simulink subsystem "In_Plane_Model"  (R2025b)
settings: Solver=VariableStepAuto  StartTime=0.0  StopTime=10.0  RelTol=1e-3
undefined symbols (not defined in the file): AeroLiftCff, AeroLongDrgCff, AeroMotoEffctArea, AeroPitchMomentCff, AeroPitchMomentLngth, AeroRltWindAngVect, AeroSideFrcCff, AeroYawMomentCff, aMode, BrkFrntBrkActrBore, BrkFrntBrkActrPrsBpt, BrkFrntBrkPadMeanRadius, BrkFrntBrkTrqTbl, BrkFrntIntrnRadius, BrkFrntKinFricCff, BrkFrntPadNum, BrkFrntShoePinToDrumCntrDst, BrkFrntShoePinToFrcAppDst, BrkFrntShoePinToPadEndAng, BrkFrntShoePinToPadStartAng, BrkFrntStcFricCff, BrkFrntWhlSpdBpt, BrkRearBrkActrBore, BrkRearBrkActrPrsBpt, BrkRearBrkPadMeanRadius, BrkRearBrkTrqTbl, BrkRearIntrnRadius, BrkRearKinFricCff, BrkRearPadNum, BrkRearShoePinToDrumCntrDst, BrkRearShoePinToFrcAppDst, BrkRearShoePinToPadEndAng, BrkRearShoePinToPadStartAng, BrkRearStcFricCff, BrkRearWhlSpdBpt, EnvAbsPrs, EnvAirTemp, FrkFrL0, FrmAng0, g, GasCnst, InitFrkLngth, InitMainFrmPitchAng, InitRearArmPitchAng, InitRearCntctPtchLatVel, InitRearCntctPtchLongVel, InitRearCntctPtchY, InitRearCntctPtchZ, InitRollAng, InitYawAng, MotoFrmLngth, MotoFrmMass, MotoGrvty, MotoLatOfst, MotoLongOfst, MotoLowrFrntFrkMass, MotoPtchOfst, MotoRearArmLngth, MotoRearArmMass, MotoRollOfst ... (+25)
libraries: sm_lib x309, nesl_utility_internal x158, nesl_utility x7, autolibsharedcoupling x6, vehdynlibtire x6, sharedtransform x4, shared6dof x1, matrix_library x1, vehdynlibeomcommon x1
(part 3 of 10)

== system In_Plane_Model/Chassis, Tires, and Areo/Chassis Body, Suspension, and Steering/CHASSIS/Chassis body/JointHubRr ==
  Bus Creator : BusCreator  Inputs=3
  PS-Simulink Converter3 : nesl_utility_internal/PS-Simulink Converter  PhysicalDomain=network_engine_domain  SubClassName=ps_output  LeftPortType=input  RightPortType=output  PseudoPeriodic=off  Frequencies=[]  VectorFormat=1-D array  Unit=inherit  AffineConversion=off
  PS-Simulink Converter4 : nesl_utility_internal/PS-Simulink Converter  PhysicalDomain=network_engine_domain  SubClassName=ps_output  LeftPortType=input  RightPortType=output  PseudoPeriodic=off  Frequencies=[]  VectorFormat=1-D array  Unit=inherit  AffineConversion=off
  PS-Simulink Converter8 : nesl_utility_internal/PS-Simulink Converter  PhysicalDomain=network_engine_domain  SubClassName=ps_output  LeftPortType=input  RightPortType=output  PseudoPeriodic=off  Frequencies=[]  VectorFormat=1-D array  Unit=inherit  AffineConversion=off
  Pitch dof : sm_lib/Joints/Revolute Joint  JointMode=Normal  CompositeWrenchDir=FollowerOnBase  CompositeWrenchFrame=BaseFrame  SenseConstraintForce=off  SenseConstraintTorque=off  SenseTotalForce=off  SenseTotalTorque=off  PositionTargetSpecify=on  PositionTargetPriority=High  PositionTargetValue=InitRearArmPitchAng  PositionTargetValueUnits=rad  VelocityTargetSpecify=on  VelocityTargetPriority=High  VelocityTargetValue=InitRearArmPitchRate  VelocityTargetValueUnits=rad/s  EquilibriumPosition=0  EquilibriumPositionUnits=rad  SpringStiffness=0  SpringStiffnessUnits=N*m/rad  DampingCoefficient=0  DampingCoefficientUnits=N*m/(rad/s)  LowerLimitSpecify=off  LowerLimitBound=-90  LowerLimitBoundUnits=deg  LowerLimitStiffness=1e4  LowerLimitStiffnessUnits=N*m/deg  LowerLimitDamping=10  LowerLimitDampingUnits=N*m/(deg/s)  LowerLimitTransitionRegionWidth=0.1  LowerLimitTransitionRegionWidthUnits=deg  UpperLimitSpecify=off  UpperLimitBound=90  UpperLimitBoundUnits=deg  UpperLimitStiffness=1e4  UpperLimitStiffnessUnits=N*m/deg  UpperLimitDamping=10  UpperLimitDampingUnits=N*m/(deg/s)  UpperLimitTransitionRegionWidth=0.1  UpperLimitTransitionRegionWidthUnits=deg  TorqueActuationMode=NoTorque  MotionActuationMode=ComputedMotion  SensePosition=on  SenseVelocity=on  SenseAcceleration=on  SenseTorqueForce=off  SenseLowerLimitTorqueForce=off  SenseUpperLimitTorqueForce=off
  World vertical frame : Subsystem  VariantControl=World vertical
  X_-pi/2 : sm_lib/Frames and Transforms/Rigid Transform  RotationMethod=StandardAxis  FollAlignAxisA=+X  BaseAlignAxisA=+Y  FollAlignAxisB=+Y  BaseAlignAxisB=+Z  RotationStandardAxis=+X  RotationAngle=-pi/2  RotationAngleUnits=rad  RotationArbitraryAxis=[0 0 1]  RotationSequenceAxes=FollowerAxes  RotationSequence=XYX  RotationSequenceAngles=[0 0 0]  RotationSequenceAnglesUnits=deg  RotationMatrix=[1 0 0; 0 1 0; 0 0 1]  Quaternion=[1 0 0 0]  TranslationMethod=None  TranslationCartesianOffset=[0 0 0]  TranslationCartesianOffsetUnits=m  TranslationStandardAxis=+Z  TranslationStandardOffset=0  TranslationStandardOffsetUnits=m  TranslationROffset=0  TranslationROffsetUnits=m  TranslationThetaOffset=0  TranslationThetaOffsetUnits=deg  TranslationZOffset=0  TranslationZOffsetUnits=m
  X_pi/2 : sm_lib/Frames and Transforms/Rigid Transform  RotationMethod=StandardAxis  FollAlignAxisA=+X  BaseAlignAxisA=+Y  FollAlignAxisB=+Y  BaseAlignAxisB=+Z  RotationStandardAxis=+X  RotationAngle=pi/2  RotationAngleUnits=rad  RotationArbitraryAxis=[0 0 1]  RotationSequenceAxes=FollowerAxes  RotationSequence=XYX  RotationSequenceAngles=[0 0 0]  RotationSequenceAnglesUnits=deg  RotationMatrix=[1 0 0; 0 1 0; 0 0 1]  Quaternion=[1 0 0 0]  TranslationMethod=None  TranslationCartesianOffset=[0 0 0]  TranslationCartesianOffsetUnits=m  TranslationStandardAxis=+Z  TranslationStandardOffset=0  TranslationStandardOffsetUnits=m  TranslationROffset=0  TranslationROffsetUnits=m  TranslationThetaOffset=0  TranslationThetaOffsetUnits=deg  TranslationZOffset=0  TranslationZOffsetUnits=m
  F : PMIOPort  Side=Left
  WVFrame_WhlRr : PMIOPort  Port=2  Side=Left
  B : PMIOPort  Port=3  Side=Right
  A,V,P : Outport
  wires:
  PS-Simulink Converter8/1 -> Bus Creator/2  "ArmRrAngV"
  Bus Creator/1 -> A,V,P/1  "ArmRrAng"
  PS-Simulink Converter3/1 -> Bus Creator/1  "ArmRrAngA"
  PS-Simulink Converter4/1 -> Bus Creator/3  "ArmRrAng"
  connections:
  WVFrame_WhlRr/RConn1 -- World vertical frame/RConn1
  X_pi/2/LConn1 -- Pitch dof/RConn1
  PS-Simulink Converter8/LConn1 -- Pitch dof/RConn3
  PS-Simulink Converter3/LConn1 -- Pitch dof/RConn4
  PS-Simulink Converter4/LConn1 -- Pitch dof/RConn2
  X_-pi/2/LConn1 -- B/RConn1
  F/RConn1 -- World vertical frame/LConn1 -- X_pi/2/RConn1
  Pitch dof/LConn1 -- X_-pi/2/RConn1

== system In_Plane_Model/Chassis, Tires, and Areo/Chassis Body, Suspension, and Steering/CHASSIS/Chassis body/Origin&Env ==
  Course shape : Subsystem  Variant=on  VariantControlMode=label  VariantControl=Choice  LabelModeActiveChoice=none
  Ground : Subsystem  Commented=on
  Inertial Frame : sm_lib/Body Elements/Graphic  Commented=on  GraphicType=Marker  MarkerShape=Frame  MarkerSize=30  GraphicVisPropType=SimpleVisualProperties  GraphicDiffuseColor=[0.0 0.0 0.0]  GraphicOpacity=1.0  GraphicSpecularColor=[0.5 0.5 0.5 1.0]  GraphicAmbientColor=[0.15 0.15 0.15 1.0]  GraphicEmissiveColor=[0.0 0.0 0.0 1.0]  GraphicShininess=75
  Mechanism Configuration : sm_lib/Utilities/Mechanism Configuration  UniformGravity=Constant  GravityVector=[-MotoGrvty*sin(0) 0 -MotoGrvty*cos(0)]  GravityVectorUnits=m/s^2  LinearizationDelta=0.001  JointModeTransitionNonlinearIterations=2
  Solver Configuration : nesl_utility_internal/Solver Configuration  PhysicalDomain=network_engine_domain  SubClassName=solver  LeftPortType=input  RightPortType=generic  Tones=[]  Harmonics=[]  SimulateNoise=off  Profile=off  UseLocalSampling=off  EnableSwitchedLinearOptims=on  FrequencyDomain=off  UseCCode=off  RelTol=0.001  AbsTol=1e-06  MinStep=1e-09  ToWorkspace=off  RevertToSquareIcSolve=off  NumHomotopyIterations=100  PhasorMode=off  PhasorModeNumHarmonics=1  ConsistencySolver=NEWTON_FTOL  IndexReductionMethod=DerivativeReplacement  DoDC=off  ResidualTolerance=1e-3  ConsistencyTolSource=GLOBAL  ConsistencyAbsTol=0.001  ConsistencyRelTol=0.001  ConsistencyTolFactor=0.001  UseLocalSolver=on  LocalSolverChoice=NE_BACKWARD_EULER_ADVANCER  ResolveIndetEquations=on  FunctionEvalNumThread=1  LocalSolverSampleTime=0.01  DoFixedCost=off  MaxNonlinIter=3  MaxModeIter=2  ComputeImpulses=off  ImpulseIterations=2  LinearAlgebra=Sparse  LinearAlgebraNumThread=0  EquationFormulation=NE_TIME_EF  DelaysMemoryBudget=1024  AutomaticFiltering=on  FilteringTimeConstant=0.001  PartitionStorageMethod=AS_NEEDED  PartitionMemoryBudget=1024  PartitionMethod=FAST  MultibodyUseLocalSolver=on  MultibodyLocalSolverChoice=ODE1  MultibodyLocalSolverSampleTime=0.01
  World Frame : sm_lib/Frames and Transforms/World Frame
  setSAE : sm_lib/Frames and Transforms/Rigid Transform  RotationMethod=StandardAxis  FollAlignAxisA=+X  BaseAlignAxisA=+Y  FollAlignAxisB=+Y  BaseAlignAxisB=+Z  RotationStandardAxis=+X  RotationAngle=pi  RotationAngleUnits=rad  RotationArbitraryAxis=[0 0 1]  RotationSequenceAxes=FollowerAxes  RotationSequence=XYX  RotationSequenceAngles=[0 0 0]  RotationSequenceAnglesUnits=deg  RotationMatrix=[1 0 0; 0 1 0; 0 0 1]  Quaternion=[1 0 0 0]  TranslationMethod=None  TranslationCartesianOffset=[0 0 0]  TranslationCartesianOffsetUnits=m  TranslationStandardAxis=+Z  TranslationStandardOffset=0  TranslationStandardOffsetUnits=m  TranslationROffset=0  TranslationROffsetUnits=m  TranslationThetaOffset=0  TranslationThetaOffsetUnits=deg  TranslationZOffset=0  TranslationZOffsetUnits=m
  F : PMIOPort  Side=Left
  connections:
  setSAE/RConn1 -- F/RConn1 -- Inertial Frame/RConn1
  Course shape/LConn1 -- Ground/LConn1 -- setSAE/LConn1 -- Solver Configuration/RConn1 -- Mechanism Configuration/RConn1 -- World Frame/RConn1

== system In_Plane_Model/Chassis, Tires, and Areo/Chassis Body, Suspension, and Steering/CHASSIS/Chassis body/mass_ArmRr ==
  CGCoord. : sm_lib/Frames and Transforms/Rigid Transform  RotationMethod=None  FollAlignAxisA=+X  BaseAlignAxisA=+Y  FollAlignAxisB=+Y  BaseAlignAxisB=+Z  RotationStandardAxis=+X  RotationAngle=0  RotationAngleUnits=rad  RotationArbitraryAxis=[0 0 1]  RotationSequenceAxes=FollowerAxes  RotationSequence=XYX  RotationSequenceAngles=[0 0 0]  RotationSequenceAnglesUnits=deg  RotationMatrix=[1 0 0; 0 1 0; 0 0 1]  Quaternion=[1 0 0 0]  TranslationMethod=Cartesian  TranslationCartesianOffset=MotoRearArmPos  TranslationCartesianOffsetUnits=m  TranslationStandardAxis=+X  TranslationStandardOffset=0  TranslationStandardOffsetUnits=m  TranslationROffset=0  TranslationROffsetUnits=m  TranslationThetaOffset=0  TranslationThetaOffsetUnits=deg  TranslationZOffset=0  TranslationZOffsetUnits=m
  CG_Solid : sm_lib/Body Elements/Spherical Solid  SphereRadius=3e-2  SphereRadiusUnits=m  ExportEntireGeometry=off  InertiaType=Custom  BasedOnType=Density  Density=1000  DensityUnits=kg/m^3  Mass=MotoRearArmMass  MassUnits=kg  CenterOfMass=[0 0 0]  CenterOfMassUnits=m  MomentsOfInertia=MotoRearArmInert  MomentsOfInertiaUnits=kg*m^2  ProductsOfInertia=[0 0 0]  ProductsOfInertiaUnits=kg*m^2  GraphicType=FromGeometry  MarkerShape=Sphere  MarkerSize=10  GraphicVisPropType=SimpleVisualProperties  GraphicDiffuseColor=[1.0 0.0 0.0]  GraphicOpacity=1.0  GraphicSpecularColor=[0.5 0.5 0.5 1.0]  GraphicAmbientColor=[0.15 0.15 0.15 1.0]  GraphicEmissiveColor=[0.0 0.0 0.0 1.0]  GraphicShininess=75  DoExposeReferenceFrame=on  SerializedFrames=<Frames/>
  Graphic : sm_lib/Body Elements/Graphic  GraphicType=Marker  MarkerShape=Frame  MarkerSize=30  GraphicVisPropType=SimpleVisualProperties  GraphicDiffuseColor=[0.0 0.0 1.0]  GraphicOpacity=1.0  GraphicSpecularColor=[0.5 0.5 0.5 1.0]  GraphicAmbientColor=[0.15 0.15 0.15 1.0]  GraphicEmissiveColor=[0.0 0.0 0.0 1.0]  GraphicShininess=75
  World vertical frame : Subsystem  VariantControl=World vertical
  B : PMIOPort  Side=Left
  CG : PMIOPort  Port=2  Side=Right
  WVFrame_ArmRr : PMIOPort  Port=3  Side=Right
  connections:
  WVFrame_ArmRr/RConn1 -- World vertical frame/RConn1
  Graphic/RConn1 -- B/RConn1 -- CGCoord./LConn1
  CG/RConn1 -- CGCoord./RConn1 -- World vertical frame/LConn1 -- CG_Solid/RConn1

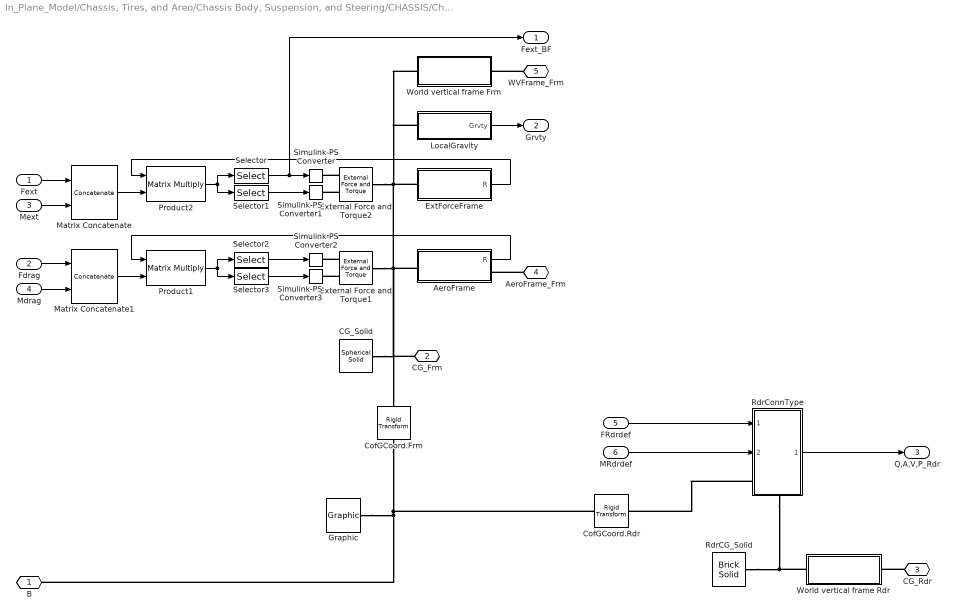
== system In_Plane_Model/Chassis, Tires, and Areo/Chassis Body, Suspension, and Steering/CHASSIS/Chassis body/mass_Frm ==
  Fext : Inport
  Fdrag : Inport  Port=2
  Mext : Inport  Port=3
  Mdrag : Inport  Port=4
  FRdrdef : Inport  Port=5
  MRdrdef : Inport  Port=6
  AeroFrame : Subsystem  Variant=on  VariantControlMode=label  VariantControl=Choice  LabelModeActiveChoice=World vertical
  CG_Solid : sm_lib/Body Elements/Spherical Solid  SphereRadius=3e-2  SphereRadiusUnits=m  ExportEntireGeometry=off  InertiaType=Custom  BasedOnType=Density  Density=1000  DensityUnits=kg/m^3  Mass=MotoFrmMass  MassUnits=kg  CenterOfMass=[0 0 0]  CenterOfMassUnits=m  MomentsOfInertia=MotoFrmInert  MomentsOfInertiaUnits=kg*m^2  ProductsOfInertia=[0 0 0]  ProductsOfInertiaUnits=kg*m^2  GraphicType=FromGeometry  MarkerShape=Sphere  MarkerSize=10  GraphicVisPropType=SimpleVisualProperties  GraphicDiffuseColor=[1.0 0.0 0.0]  GraphicOpacity=1.0  GraphicSpecularColor=[0.5 0.5 0.5 1.0]  GraphicAmbientColor=[0.15 0.15 0.15 1.0]  GraphicEmissiveColor=[0.0 0.0 0.0 1.0]  GraphicShininess=75  DoExposeReferenceFrame=on  SerializedFrames=<Frames/>
  CofGCoord.Frm : sm_lib/Frames and Transforms/Rigid Transform  RotationMethod=None  FollAlignAxisA=+X  BaseAlignAxisA=+Y  FollAlignAxisB=+Y  BaseAlignAxisB=+Z  RotationStandardAxis=+X  RotationAngle=0  RotationAngleUnits=rad  RotationArbitraryAxis=[0 0 1]  RotationSequenceAxes=FollowerAxes  RotationSequence=XYX  RotationSequenceAngles=[0 0 0]  RotationSequenceAnglesUnits=deg  RotationMatrix=[1 0 0; 0 1 0; 0 0 1]  Quaternion=[1 0 0 0]  TranslationMethod=Cartesian  TranslationCartesianOffset=MotoFrmCm  TranslationCartesianOffsetUnits=m  TranslationStandardAxis=+X  TranslationStandardOffset=0  TranslationStandardOffsetUnits=m  TranslationROffset=0  TranslationROffsetUnits=m  TranslationThetaOffset=0  TranslationThetaOffsetUnits=deg  TranslationZOffset=0  TranslationZOffsetUnits=m
  CofGCoord.Rdr : sm_lib/Frames and Transforms/Rigid Transform  RotationMethod=None  FollAlignAxisA=+X  BaseAlignAxisA=+Y  FollAlignAxisB=+Y  BaseAlignAxisB=+Z  RotationStandardAxis=+X  RotationAngle=0  RotationAngleUnits=rad  RotationArbitraryAxis=[0 0 1]  RotationSequenceAxes=FollowerAxes  RotationSequence=XYX  RotationSequenceAngles=[0 0 0]  RotationSequenceAnglesUnits=deg  RotationMatrix=[1 0 0; 0 1 0; 0 0 1]  Quaternion=[1 0 0 0]  TranslationMethod=Cartesian  TranslationCartesianOffset=RiderCmLoct  TranslationCartesianOffsetUnits=m  TranslationStandardAxis=+X  TranslationStandardOffset=0  TranslationStandardOffsetUnits=m  TranslationROffset=0  TranslationROffsetUnits=m  TranslationThetaOffset=0  TranslationThetaOffsetUnits=deg  TranslationZOffset=0  TranslationZOffsetUnits=m
  ExtForceFrame : Subsystem  Variant=on  VariantControlMode=label  VariantControl=Choice  LabelModeActiveChoice=World vertical
  External Force and Torque1 : sm_lib/Forces and Torques/External Force and Torque  EnableForceX=off  EnableForceY=off  EnableForceZ=off  EnableForce=on  ForceResolutionFrame=AttachedFrame  EnableTorqueX=off  EnableTorqueY=off  EnableTorqueZ=off  EnableTorque=on  TorqueResolutionFrame=AttachedFrame
  External Force and Torque2 : sm_lib/Forces and Torques/External Force and Torque  EnableForceX=off  EnableForceY=off  EnableForceZ=off  EnableForce=on  ForceResolutionFrame=AttachedFrame  EnableTorqueX=off  EnableTorqueY=off  EnableTorqueZ=off  EnableTorque=on  TorqueResolutionFrame=AttachedFrame
  Graphic : sm_lib/Body Elements/Graphic  GraphicType=Marker  MarkerShape=Frame  MarkerSize=30  GraphicVisPropType=SimpleVisualProperties  GraphicDiffuseColor=[0.0 0.0 1.0]  GraphicOpacity=1.0  GraphicSpecularColor=[0.5 0.5 0.5 1.0]  GraphicAmbientColor=[0.15 0.15 0.15 1.0]  GraphicEmissiveColor=[0.0 0.0 0.0 1.0]  GraphicShininess=75
  LocalGravity : Subsystem
  Matrix Concatenate : Concatenate  Mode=Multidimensional array  ConcatenateDimension=2
  Matrix Concatenate1 : Concatenate  Mode=Multidimensional array  ConcatenateDimension=2
  Product1 : Product  Multiplication=Matrix(*)
  Product2 : Product  Multiplication=Matrix(*)
  RdrCG_Solid : sm_lib/Body Elements/Brick Solid  BrickDimensions=[1 1 1]*0.1  BrickDimensionsUnits=m  ExportEntireGeometry=off  InertiaType=Custom  BasedOnType=Density  Density=1000  DensityUnits=kg/m^3  Mass=RiderMass  MassUnits=kg  CenterOfMass=[0 0 0]  CenterOfMassUnits=m  MomentsOfInertia=RiderInert  MomentsOfInertiaUnits=kg*m^2  ProductsOfInertia=[0 0 0]  ProductsOfInertiaUnits=kg*m^2  GraphicType=FromGeometry  MarkerShape=Sphere  MarkerSize=10  GraphicVisPropType=SimpleVisualProperties  GraphicDiffuseColor=[0.4 0.4 0.4]  GraphicOpacity=1.0  GraphicSpecularColor=[0.5 0.5 0.5 1.0]  GraphicAmbientColor=[0.15 0.15 0.15 1.0]  GraphicEmissiveColor=[0.0 0.0 0.0 1.0]  GraphicShininess=75  DoExposeReferenceFrame=on  SerializedFrames=<Frames/>
  RdrConnType : Subsystem  Variant=on  VariantChoicesSpecifier={'Rigid', 's6DOF_and_External_Forces_and_Moments'}  VariantControlMode=label  VariantControl=Choice  LabelModeActiveChoice=Rigid
      settings: PortSchema="{\"entries\":[{\"content\":{\"sides\":[{\"content\":{\"connectorIds\":[\"In1\",\"In2\",\"LConn1\"]},\"type\":\"ConnectorPlacement.EquallySpacedRectSide\",\"uuid\":\"6027bf0c-47dc-4641-b312-91f0cbb185cc\"},{\"content\":{\"connectorIds\":[\"Out1\"],\"side\":\"RIGHT\"},\"type\":\"ConnectorPlacement.EquallySpacedRectSide\",\"uuid\":\"75561f8d-b6fc-4ce9-bdf9-6e985548130f\"},{\"content\":{\"side\":\"TOP\"},\"type\":\"ConnectorPlacement.EquallySpacedRectSide\",\"uuid\":\"398f9736-f514-4440-baa3-55debf119b8f\"},{\"content\":{\"connectorIds\":[\"RConn1\"],\"side\":\"BOTTOM\"},\"type\":\"ConnectorPlacement.EquallySpacedRectSide\",\"uuid\":\"dfd8777e-2555-41c1-b77e-3f19d71f018f\"}]},\"type\":\"ConnectorPlacement.EquallySpacedConnector\",\"uuid\":\"9426d2e3-04b5-4679-a13c-19ca1f9bfd84\"}],\"packageUris\":[\"http://schema.mathworks.com/mf0/Connector/R2020b\"],\"version\":\"1.0\"}"
  Selector : Selector  NumberOfDimensions=2  InputPortWidth=3  IndexOptions=Index vector (dialog),Index vector (dialog)  Indices=[1 2 3],[1]  OutputSizes=1,1
  Selector1 : Selector  NumberOfDimensions=2  InputPortWidth=3  IndexOptions=Index vector (dialog),Index vector (dialog)  Indices=[1 2 3],[2]  OutputSizes=1,1
  Selector2 : Selector  NumberOfDimensions=2  InputPortWidth=3  IndexOptions=Index vector (dialog),Index vector (dialog)  Indices=[1 2 3],[1]  OutputSizes=1,1
  Selector3 : Selector  NumberOfDimensions=2  InputPortWidth=3  IndexOptions=Index vector (dialog),Index vector (dialog)  Indices=[1 2 3],[2]  OutputSizes=1,1
  Simulink-PS Converter : nesl_utility_internal/Simulink-PS Converter  PhysicalDomain=network_engine_domain  SubClassName=ps_input  LeftPortType=input  RightPortType=output  PseudoPeriodic=off  Frequencies=[]  NoiseDistribution=none  NoiseParameters=[]  Unit=N  AffineConversion=off  FilteringAndDerivatives=provide  SimscapeFilterOrder=1  InputFilterTimeConstant=0.001  UdotUserProvided=0
  Simulink-PS Converter1 : nesl_utility_internal/Simulink-PS Converter  PhysicalDomain=network_engine_domain  SubClassName=ps_input  LeftPortType=input  RightPortType=output  PseudoPeriodic=off  Frequencies=[]  NoiseDistribution=none  NoiseParameters=[]  Unit=N*m  AffineConversion=off  FilteringAndDerivatives=provide  SimscapeFilterOrder=1  InputFilterTimeConstant=0.001  UdotUserProvided=0
  Simulink-PS Converter2 : nesl_utility_internal/Simulink-PS Converter  PhysicalDomain=network_engine_domain  SubClassName=ps_input  LeftPortType=input  RightPortType=output  PseudoPeriodic=off  Frequencies=[]  NoiseDistribution=none  NoiseParameters=[]  Unit=N  AffineConversion=off  FilteringAndDerivatives=provide  SimscapeFilterOrder=1  InputFilterTimeConstant=0.001  UdotUserProvided=0
  Simulink-PS Converter3 : nesl_utility_internal/Simulink-PS Converter  PhysicalDomain=network_engine_domain  SubClassName=ps_input  LeftPortType=input  RightPortType=output  PseudoPeriodic=off  Frequencies=[]  NoiseDistribution=none  NoiseParameters=[]  Unit=N*m  AffineConversion=off  FilteringAndDerivatives=provide  SimscapeFilterOrder=1  InputFilterTimeConstant=0.001  UdotUserProvided=0
  World vertical frame Frm : Subsystem  VariantControl=World vertical
  World vertical frame Rdr : Subsystem  VariantControl=World vertical
  B : PMIOPort  Side=Left
  CG_Frm : PMIOPort  Port=2  Side=Right
  CG_Rdr : PMIOPort  Port=3  Side=Right
  AeroFrame_Frm : PMIOPort  Port=4  Side=Right
  WVFrame_Frm : PMIOPort  Port=5  Side=Right
  Fext_BF : Outport
  Grvty : Outport  Port=2
  Q,A,V,P_Rdr : Outport  Port=3
  wires:
  FRdrdef/1 -> RdrConnType/1(FRdrdef)
  MRdrdef/1 -> RdrConnType/2(MRdrdef)
  RdrConnType/1(Q,A,V,P_Rdr) -> Q,A,V,P_Rdr/1
  AeroFrame/1(R) -> Product1/1
  Fdrag/1 -> Matrix Concatenate1/1
  Mdrag/1 -> Matrix Concatenate1/2
  Selector3/1 -> Simulink-PS Converter3/1
  Matrix Concatenate1/1 -> Product1/2
  Product1/1 -> Selector3/1, Selector2/1
  Selector2/1 -> Simulink-PS Converter2/1
  LocalGravity/1(Grvty) -> Grvty/1
  Selector/1 -> Fext_BF/1, Simulink-PS Converter/1
  Product2/1 -> Selector/1, Selector1/1
  Matrix Concatenate/1 -> Product2/2
  Selector1/1 -> Simulink-PS Converter1/1
  Mext/1 -> Matrix Concatenate/2
  Fext/1 -> Matrix Concatenate/1
  ExtForceFrame/1(R) -> Product2/1
  connections:
  CG_Rdr/RConn1 -- World vertical frame Rdr/RConn1
  WVFrame_Frm/RConn1 -- World vertical frame Frm/RConn1
  AeroFrame_Frm/RConn1 -- AeroFrame/RConn1
  RdrConnType/LConn1 -- CofGCoord.Rdr/RConn1
  World vertical frame Rdr/LConn1 -- RdrConnType/RConn1 -- RdrCG_Solid/RConn1
  External Force and Torque1/LConn1 -- Simulink-PS Converter2/RConn1
  External Force and Torque1/LConn2 -- Simulink-PS Converter3/RConn1
  ExtForceFrame/LConn1 -- External Force and Torque1/RConn1 -- AeroFrame/LConn1 -- CG_Frm/RConn1 -- CofGCoord.Frm/RConn1 -- CG_Solid/RConn1 -- LocalGravity/LConn1 -- World vertical frame Frm/LConn1 -- External Force and Torque2/RConn1
  External Force and Torque2/LConn2 -- Simulink-PS Converter1/RConn1
  External Force and Torque2/LConn1 -- Simulink-PS Converter/RConn1
  CofGCoord.Frm/LConn1 -- CofGCoord.Rdr/LConn1 -- B/RConn1 -- Graphic/RConn1

== system In_Plane_Model/Chassis, Tires, and Areo/Chassis Body, Suspension, and Steering/CHASSIS/Chassis body/pivo (dofPitch) ==
  MSusr : Inport
  Bus Creator : BusCreator  Inputs=3
  Selector : Selector  InputPortWidth=3  IndexOptions=Index vector (dialog)  Indices=3  OutputSizes=1
  pivo : Subsystem  Variant=on  VariantControlMode=label  VariantControl=Choice  LabelModeActiveChoice=pivo
  B : PMIOPort  Side=Left
  F : PMIOPort  Port=2  Side=Left
  A,V,P : Outport
  My : Outport  Port=2
  wires:
  MSusr/1 -> pivo/1(t)
  Bus Creator/1 -> A,V,P/1  "FrmAng"
  pivo/1(q) -> Bus Creator/3  "FrmAng"
  pivo/3(b) -> Bus Creator/1  "FrmAngA"
  pivo/2(w) -> Bus Creator/2  "FrmAngV"
  Selector/1 -> My/1  "MsuspRr"
  pivo/4(tt) -> Selector/1
  connections:
  pivo/RConn1 -- F/RConn1
  pivo/LConn1 -- B/RConn1

== system In_Plane_Model/Chassis, Tires, and Areo/Chassis Body, Suspension, and Steering/CHASSIS/Sensors/Geom sensor ==
  Bus Creator : BusCreator  Inputs=12
  Graphic1 : sm_lib/Body Elements/Graphic  GraphicType=Marker  MarkerShape=Frame  MarkerSize=20  GraphicVisPropType=SimpleVisualProperties  GraphicDiffuseColor=[1 1 0]  GraphicOpacity=1.0  GraphicSpecularColor=[0.5 0.5 0.5 1.0]  GraphicAmbientColor=[0.15 0.15 0.15 1.0]  GraphicEmissiveColor=[0.0 0.0 0.0 1.0]  GraphicShininess=75
  Graphic2 : sm_lib/Body Elements/Graphic  GraphicType=Marker  MarkerShape=Frame  MarkerSize=20  GraphicVisPropType=SimpleVisualProperties  GraphicDiffuseColor=[1 1 0]  GraphicOpacity=1.0  GraphicSpecularColor=[0.5 0.5 0.5 1.0]  GraphicAmbientColor=[0.15 0.15 0.15 1.0]  GraphicEmissiveColor=[0.0 0.0 0.0 1.0]  GraphicShininess=75
  Graphic3 : sm_lib/Body Elements/Graphic  GraphicType=Marker  MarkerShape=Frame  MarkerSize=20  GraphicVisPropType=SimpleVisualProperties  GraphicDiffuseColor=[1 1 0]  GraphicOpacity=1.0  GraphicSpecularColor=[0.5 0.5 0.5 1.0]  GraphicAmbientColor=[0.15 0.15 0.15 1.0]  GraphicEmissiveColor=[0.0 0.0 0.0 1.0]  GraphicShininess=75
  Sensor_HubFr : Subsystem
  Sensor_HubRr : Subsystem
  Sensor_origin : Subsystem
  UE4orig2HubFr : sm_lib/Frames and Transforms/Rigid Transform  RotationMethod=None  FollAlignAxisA=+X  BaseAlignAxisA=+Y  FollAlignAxisB=+Y  BaseAlignAxisB=+Z  RotationStandardAxis=+X  RotationAngle=0  RotationAngleUnits=rad  RotationArbitraryAxis=[0 0 1]  RotationSequenceAxes=FollowerAxes  RotationSequence=XYX  RotationSequenceAngles=[0 0 0]  RotationSequenceAnglesUnits=deg  RotationMatrix=[1 0 0; 0 1 0; 0 0 1]  Quaternion=[1 0 0 0]  TranslationMethod=Cartesian  TranslationCartesianOffset=[ScnFrntHubX, 0, ScnFrntHubZ]  TranslationCartesianOffsetUnits=m  TranslationStandardAxis=+X  TranslationStandardOffset=0  TranslationStandardOffsetUnits=m  TranslationROffset=0  TranslationROffsetUnits=m  TranslationThetaOffset=0  TranslationThetaOffsetUnits=deg  TranslationZOffset=0  TranslationZOffsetUnits=m
  UE4orig2HubRr : sm_lib/Frames and Transforms/Rigid Transform  RotationMethod=None  FollAlignAxisA=+X  BaseAlignAxisA=+Y  FollAlignAxisB=+Y  BaseAlignAxisB=+Z  RotationStandardAxis=+X  RotationAngle=0  RotationAngleUnits=rad  RotationArbitraryAxis=[0 0 1]  RotationSequenceAxes=FollowerAxes  RotationSequence=XYX  RotationSequenceAngles=[0 0 0]  RotationSequenceAnglesUnits=deg  RotationMatrix=[1 0 0; 0 1 0; 0 0 1]  Quaternion=[1 0 0 0]  TranslationMethod=Cartesian  TranslationCartesianOffset=[ScnRearHubX, 0, ScnRearHubZ]  TranslationCartesianOffsetUnits=m  TranslationStandardAxis=+X  TranslationStandardOffset=0  TranslationStandardOffsetUnits=m  TranslationROffset=0  TranslationROffsetUnits=m  TranslationThetaOffset=0  TranslationThetaOffsetUnits=deg  TranslationZOffset=0  TranslationZOffsetUnits=m
  pivo2UE4orig_trans : sm_lib/Frames and Transforms/Rigid Transform  RotationMethod=None  FollAlignAxisA=+X  BaseAlignAxisA=+Y  FollAlignAxisB=+Y  BaseAlignAxisB=+Z  RotationStandardAxis=+X  RotationAngle=0  RotationAngleUnits=rad  RotationArbitraryAxis=[0 0 1]  RotationSequenceAxes=FollowerAxes  RotationSequence=XYX  RotationSequenceAngles=[0 0 0]  RotationSequenceAnglesUnits=deg  RotationMatrix=[1 0 0; 0 1 0; 0 0 1]  Quaternion=[1 0 0 0]  TranslationMethod=Cartesian  TranslationCartesianOffset=[ScnOrgnX, 0, ScnOrgnZ]  TranslationCartesianOffsetUnits=m  TranslationStandardAxis=+X  TranslationStandardOffset=0  TranslationStandardOffsetUnits=m  TranslationROffset=0  TranslationROffsetUnits=m  TranslationThetaOffset=0  TranslationThetaOffsetUnits=deg  TranslationZOffset=0  TranslationZOffsetUnits=m
  pivo2world_rot : sm_lib/Frames and Transforms/Rigid Transform  RotationMethod=StandardAxis  FollAlignAxisA=+X  BaseAlignAxisA=+Y  FollAlignAxisB=+Y  BaseAlignAxisB=+Z  RotationStandardAxis=+Y  RotationAngle=-(InitRearArmPitchAng+InitMainFrmPitchAng)  RotationAngleUnits=rad  RotationArbitraryAxis=[0 0 1]  RotationSequenceAxes=FollowerAxes  RotationSequence=XYX  RotationSequenceAngles=[0 0 0]  RotationSequenceAnglesUnits=deg  RotationMatrix=[1 0 0; 0 1 0; 0 0 1]  Quaternion=[1 0 0 0]  TranslationMethod=None  TranslationCartesianOffset=[0, 0, 0]  TranslationCartesianOffsetUnits=m  TranslationStandardAxis=+X  TranslationStandardOffset=0  TranslationStandardOffsetUnits=m  TranslationROffset=0  TranslationROffsetUnits=m  TranslationThetaOffset=0  TranslationThetaOffsetUnits=deg  TranslationZOffset=0  TranslationZOffsetUnits=m
  HubRr : PMIOPort  Side=Left
  HubFr : PMIOPort  Port=2  Side=Left
  pivo : PMIOPort  Port=3  Side=Left
  GeomInfo : Outport
  wires:
  Bus Creator/1 -> GeomInfo/1  "GeonInfo"
  Sensor_origin/1(psi) -> Bus Creator/7  "UE4orig_psi"
  Sensor_HubRr/2(y) -> Bus Creator/2  "UE4HubRr_y"
  Sensor_origin/4(x) -> Bus Creator/10  "UE4orig_x"
  Sensor_HubFr/2(y) -> Bus Creator/5  "UE4HubFr_y"
  Sensor_origin/5(y) -> Bus Creator/11  "UE4orig_y"
  Sensor_origin/2(theta) -> Bus Creator/8  "UE4orig_theta"
  Sensor_HubRr/3(z) -> Bus Creator/3  "UE4HubRr_z"
  Sensor_origin/6(z) -> Bus Creator/12  "UE4orig_z"
  Sensor_HubRr/1(x) -> Bus Creator/1  "UE4HubRr_x"
  Sensor_origin/3(phi) -> Bus Creator/9  "UE4orig_phi"
  Sensor_HubFr/1(x) -> Bus Creator/4  "UE4HubFr_x"
  Sensor_HubFr/3(z) -> Bus Creator/6  "UE4HubFr_z"
  connections:
  HubRr/RConn1 -- Sensor_HubRr/LConn2
  pivo2world_rot/LConn1 -- pivo/RConn1
  UE4orig2HubRr/RConn1 -- Sensor_HubRr/LConn1 -- Graphic1/RConn1
  Graphic3/RConn1 -- Sensor_HubFr/LConn1 -- UE4orig2HubFr/RConn1
  pivo2UE4orig_trans/LConn1 -- pivo2world_rot/RConn1
  Sensor_HubFr/LConn2 -- HubFr/RConn1
  pivo2UE4orig_trans/RConn1 -- UE4orig2HubFr/LConn1 -- Sensor_origin/LConn1 -- Graphic2/RConn1 -- UE4orig2HubRr/LConn1

== system In_Plane_Model/Chassis, Tires, and Areo/Chassis Body, Suspension, and Steering/CHASSIS/Sensors/HubFr_sensor ==
  Bus Creator2 : BusCreator  Inputs=3
  Bus Creator3 : BusCreator  Inputs=3
  Bus Creator4 : BusCreator  Inputs=3
  FrontTireRadius [m] : Bias  Bias=TireFrntWhlRadius  SaturateOnIntegerOverflow=off
  Origin : Subsystem
  PS-Simulink Converter{1..9} (9 alike) : nesl_utility_internal/PS-Simulink Converter  PhysicalDomain=network_engine_domain  SubClassName=ps_output  LeftPortType=input  RightPortType=output  PseudoPeriodic=off  Frequencies=[]  VectorFormat=1-D array  Unit=inherit  AffineConversion=off
  Transform Sensor : sm_lib/Frames and Transforms/Transform Sensor  MeasurementFrame=NonRotatingBase  RotationSequence=XYX  SenseAngle=off  SenseAxis=off  SenseQ=off  SenseR=off  SenseRotationSequence=off  SenseOmegaX=off  SenseOmegaY=off  SenseOmegaZ=off  SenseOmega=off  SenseQDot=off  SenseRDot=off  SenseRotationSequenceDot=off  SenseAlphaX=off  SenseAlphaY=off  SenseAlphaZ=off  SenseAlpha=off  SenseQDDot=off  SenseRDDot=off  SenseX=on  SenseY=on  SenseZ=on  SenseXYZ=off  SenseRad=off  SenseAzim=off  SenseDist=off  SenseInc=off  SenseXDot=on  SenseYDot=on  SenseZDot=on  SenseXYZDot=off  SenseRadDot=off  SenseAzimDot=off  SenseDistDot=off  SenseIncDot=off  SenseXDDot=on  SenseYDDot=on  SenseZDDot=on  SenseXYZDDot=off  SenseRadDDot=off  SenseAzimDDot=off  SenseDistDDot=off  SenseIncDDot=off
  World vertical frame : Subsystem  VariantControl=World vertical
  F : PMIOPort  Side=Left
  WVFrame_WhlFr : PMIOPort  Port=2  Side=Right
  A,V,P_X : Outport
  A,V,P_Y : Outport  Port=2
  A,V,P_Z : Outport  Port=3
  wires:
  FrontTireRadius [m]/1 -> Bus Creator3/3  "WhlFrCpPz"
  PS-Simulink Converter4/1 -> Bus Creator4/2  "WhlFrCpVy"
  PS-Simulink Converter5/1 -> Bus Creator2/3  "WhlFrCpPx"
  PS-Simulink Converter6/1 -> Bus Creator2/2  "WhlFrCpVx"
  PS-Simulink Converter8/1 -> Bus Creator2/1  "WhlFrCpAx"
  PS-Simulink Converter7/1 -> Bus Creator4/3  "WhlFrCpPy"
  PS-Simulink Converter2/1 -> FrontTireRadius [m]/1
  PS-Simulink Converter9/1 -> Bus Creator4/1  "WhlFrCpAy"
  PS-Simulink Converter1/1 -> Bus Creator3/2  "WhlFrCpVz"
  PS-Simulink Converter3/1 -> Bus Creator3/1  "WhlFrCpAz"
  Bus Creator4/1 -> A,V,P_Y/1  "WhlFrCpY"
  Bus Creator3/1 -> A,V,P_Z/1  "WhlFrCpZ"
  Bus Creator2/1 -> A,V,P_X/1  "WhlFrCpX"
  connections:
  World vertical frame/RConn1 -- WVFrame_WhlFr/RConn1
  Origin/RConn1 -- Transform Sensor/LConn1
  PS-Simulink Converter7/LConn1 -- Transform Sensor/RConn5
  Transform Sensor/RConn9 -- PS-Simulink Converter1/LConn1
  F/RConn1 -- World vertical frame/LConn1 -- Transform Sensor/RConn1
  PS-Simulink Converter9/LConn1 -- Transform Sensor/RConn7
  Transform Sensor/RConn2 -- PS-Simulink Converter5/LConn1
  PS-Simulink Converter8/LConn1 -- Transform Sensor/RConn4
  PS-Simulink Converter4/LConn1 -- Transform Sensor/RConn6
  Transform Sensor/RConn3 -- PS-Simulink Converter6/LConn1
  Transform Sensor/RConn8 -- PS-Simulink Converter2/LConn1
  Transform Sensor/RConn10 -- PS-Simulink Converter3/LConn1

== system In_Plane_Model/Chassis, Tires, and Areo/Chassis Body, Suspension, and Steering/CHASSIS/Steering and fork/Fork ==
  FSusf : Inport
  fork (dofPrism) : Subsystem
  mass_FrkLw : Subsystem
  mass_FrkUp : Subsystem
  offset : Subsystem
  B : PMIOPort  Side=Left
  CG_FrkLw : PMIOPort  Port=2  Side=Right
  WVFrame_FrkLw : PMIOPort  Port=3  Side=Right
  WVFrame_FrkUp : PMIOPort  Port=4  Side=Right
  F : PMIOPort  Port=5  Side=Right
  FrkFz : Outport
  Lfrk : Outport  Port=2
  wires:
  FSusf/1 -> fork (dofPrism)/1(f)
  fork (dofPrism)/1(Lfrk) -> Lfrk/1  "Lfrk"
  fork (dofPrism)/2(FrkFz) -> FrkFz/1  "FrkFz"
  connections:
  mass_FrkUp/RConn1 -- WVFrame_FrkUp/RConn1
  mass_FrkLw/RConn2 -- WVFrame_FrkLw/RConn1
  mass_FrkLw/RConn1 -- CG_FrkLw/RConn1
  mass_FrkLw/LConn1 -- offset/LConn1 -- fork (dofPrism)/RConn1
  offset/RConn1 -- F/RConn1
  fork (dofPrism)/LConn1 -- B/RConn1 -- mass_FrkUp/LConn1

== system In_Plane_Model/Chassis, Tires, and Areo/Chassis Body, Suspension, and Steering/CHASSIS/Steering and fork/Steering ==
  t : Inport
  tExt : Inport  Port=2
  MStrDmpin : Inport  Port=3
  Add : Sum  Inputs=++-
  Bus Creator : BusCreator  Inputs=3
  Steering damper : Subsystem  Variant=on  VariantChoicesSpecifier={'External_Damper', 'No_Damper', 'Simple_Damper'}  VariantControlMode=label  VariantControl=Choice  LabelModeActiveChoice=No_Damper
  Str dof : Subsystem  Variant=on  VariantChoicesSpecifier={'No_Steering', 'Steering'}  VariantControlMode=label  VariantControl=Choice  LabelModeActiveChoice=No_Steering
      settings: PortSchema="{\"entries\":[{\"content\":{\"sides\":[{\"content\":{\"connectorIds\":[\"LConn1\",\"In1\"]},\"type\":\"ConnectorPlacement.EquallySpacedRectSide\",\"uuid\":\"551717c8-8743-4e9e-b47f-5b4b103cfc62\"},{\"content\":{\"connectorIds\":[\"RConn1\",\"Out1\",\"Out2\",\"Out3\"],\"side\":\"RIGHT\"},\"type\":\"ConnectorPlacement.EquallySpacedRectSide\",\"uuid\":\"74f860b9-2276-4049-a768-37112b7d7a8f\"},{\"content\":{\"side\":\"TOP\"},\"type\":\"ConnectorPlacement.EquallySpacedRectSide\",\"uuid\":\"53392327-2051-46ae-87ba-bb6cc5758e8c\"}]},\"type\":\"ConnectorPlacement.EquallySpacedConnector\",\"uuid\":\"2a3bb02d-466e-4ec6-8c34-c3cd89ffd768\"}],\"packageUris\":[\"http://schema.mathworks.com/mf0/Connector/R2020b\"],\"version\":\"1.0\"}"
  B : PMIOPort  Side=Left
  F : PMIOPort  Port=2  Side=Right
  A,V,P : Outport
  wires:
  tExt/1 -> Add/2
  MStrDmpin/1 -> Steering damper/2(MStrDmpin)
  Steering damper/1(MStrDmp) -> Add/3
  Add/1 -> Str dof/1(t)
  t/1 -> Add/1
  Str dof/3(q) -> Bus Creator/3  "StrAng"
  Bus Creator/1 -> A,V,P/1  "FrmAng"
  Str dof/1(b) -> Bus Creator/1  "StrAngA"
  Str dof/2(w) -> Steering damper/1(StrAngV), Bus Creator/2  "StrAngV"
  connections:
  Str dof/RConn1 -- F/RConn1
  Str dof/LConn1 -- B/RConn1

== system In_Plane_Model/Chassis, Tires, and Areo/Chassis Body, Suspension, and Steering/CHASSIS/Suspension F&M/FrSus F&M ==
  note: 1) Add Subsystem or Model blocks as valid variant choices.
      | 2) You cannot connect blocks at this level. At simulation, connectivity is automatically
      | determined, based on the active variant and port name matching.
  Lfrk : Inport
  FSusfin : Inport  Port=2
  External_Suspension : Subsystem  VariantControl=External_Suspension  ReferencedSubsystem=External_Suspension
  Simple_Spring_and_Damper_Suspension : Subsystem  VariantControl=Simple_Spring_and_Damper_Suspension  ReferencedSubsystem=Simple_Spring_and_Damper_Suspension
  FSusf : Outport

== system In_Plane_Model/Chassis, Tires, and Areo/Chassis Body, Suspension, and Steering/CHASSIS/Suspension F&M/RrSus F&M ==
  note: 1) Add Subsystem or Model blocks as valid variant choices.
      | 2) You cannot connect blocks at this level. At simulation, connectivity is automatically
      | determined, based on the active variant and port name matching.
  Frm : Inport
  MSusrin : Inport  Port=2
  External_Suspension2 : Subsystem  VariantControl=External_Suspension2  ReferencedSubsystem=External_Suspension2
  Simple_Spring_and_Damper_Suspension2 : Subsystem  VariantControl=Simple_Spring_and_Damper_Suspension2  ReferencedSubsystem=Simple_Spring_and_Damper_Suspension2
  MSusf : Outport

== system In_Plane_Model/Chassis, Tires, and Areo/Chassis Body, Suspension, and Steering/Signal routine/Ancillary_sub/Velocities ==
  Bus Creator6 : BusCreator  Inputs=21
  Sensor : Subsystem
  WVFrame_WhlRr : PMIOPort  Side=Left
  WVFrame_WhlFr : PMIOPort  Port=2  Side=Left
  WVFrame_ArmRr : PMIOPort  Port=3  Side=Left
  WVFrame_FrkUp : PMIOPort  Port=4  Side=Left
  WVFrame_FrkLw : PMIOPort  Port=5  Side=Left
  WVFrame_Rdr : PMIOPort  Port=6  Side=Left
  WVFrame_Frm : PMIOPort  Port=7  Side=Left
  vel : Outport
  wires:
  Sensor/5(RdrVx) -> Bus Creator6/5
  Sensor/12(RdrVy) -> Bus Creator6/12
  Sensor/19(RdrVz) -> Bus Creator6/19
  Sensor/21(FrkLwVz) -> Bus Creator6/21
  Sensor/20(FrkUpVz) -> Bus Creator6/20
  Sensor/18(FrmVz) -> Bus Creator6/18
  Sensor/17(ArmRrVz) -> Bus Creator6/17
  Sensor/16(WhlFrVz) -> Bus Creator6/16
  Sensor/15(WhlRrVz) -> Bus Creator6/15
  Sensor/14(FrkLwVy) -> Bus Creator6/14
  Sensor/13(FrkUpVy) -> Bus Creator6/13
  Sensor/11(FrmVy) -> Bus Creator6/11
  Sensor/10(ArmRrVy) -> Bus Creator6/10
  Sensor/9(WhlFrVy) -> Bus Creator6/9
  Sensor/8(WhlRrVy) -> Bus Creator6/8
  Sensor/7(FrkLwVx) -> Bus Creator6/7
  Sensor/6(FrkUpVx) -> Bus Creator6/6
  Sensor/4(FrmVx) -> Bus Creator6/4
  Sensor/3(ArmRrVx) -> Bus Creator6/3
  Sensor/2(WhlFrVx) -> Bus Creator6/2
  Sensor/1(WhlRrVx) -> Bus Creator6/1
  Bus Creator6/1 -> vel/1  "Vel"
  connections:
  Sensor/LConn4 -- WVFrame_Frm/RConn1
  WVFrame_Rdr/RConn1 -- Sensor/LConn5
  Sensor/LConn7 -- WVFrame_FrkLw/RConn1
  Sensor/LConn6 -- WVFrame_FrkUp/RConn1
  Sensor/LConn3 -- WVFrame_ArmRr/RConn1
  Sensor/LConn2 -- WVFrame_WhlFr/RConn1
  WVFrame_WhlRr/RConn1 -- Sensor/LConn1

== system In_Plane_Model/Chassis, Tires, and Areo/Chassis Body, Suspension, and Steering/Signal routine/Geom/FrmRotInfo ==
  psi : Inport
  theta : Inport  Port=2
  phi : Inport  Port=3
  Bias1 : Bias  Bias=MotoYawOfst  SaturateOnIntegerOverflow=off
  Bias2 : Bias  Bias=MotoRollOfst  SaturateOnIntegerOverflow=off
  Bias3 : Bias  Bias=MotoPtchOfst  SaturateOnIntegerOverflow=off
  Rotation : Concatenate  NumInputs=3  Mode=Multidimensional array  ConcatenateDimension=2
  phi theta psi : Outport
  wires:
  phi/1 -> Bias2/1
  psi/1 -> Bias1/1
  theta/1 -> Bias3/1
  Bias3/1 -> Rotation/2
  Rotation/1 -> phi theta psi/1
  Bias2/1 -> Rotation/1
  Bias1/1 -> Rotation/3

== system In_Plane_Model/Chassis, Tires, and Areo/Chassis Body, Suspension, and Steering/Signal routine/Geom/StrRotInfo ==
  delta : Inport
  Bias2 : Bias  Bias=MotoStrgOfst  SaturateOnIntegerOverflow=off
  Constant : Constant  Value=0
  Constant1 : Constant  Value=0
  Frame1 : Concatenate  NumInputs=3  Mode=Multidimensional array  ConcatenateDimension=2
  AngStr : Outport
  wires:
  Constant/1 -> Frame1/1
  Frame1/1 -> AngStr/1  "Whl"
  Bias2/1 -> Frame1/3
  Constant1/1 -> Frame1/2
  delta/1 -> Bias2/1

== system In_Plane_Model/Chassis, Tires, and Areo/Chassis Body, Suspension, and Steering/Signal routine/Geom/posFw_l ==
  x : Inport
  y : Inport  Port=2
  z : Inport  Port=3
  Frame1 : Concatenate  NumInputs=3  Mode=Multidimensional array  ConcatenateDimension=2
  xyz : Outport
  wires:
  Frame1/1 -> xyz/1
  z/1 -> Frame1/3
  x/1 -> Frame1/1
  y/1 -> Frame1/2

== system In_Plane_Model/Chassis, Tires, and Areo/Chassis Body, Suspension, and Steering/Signal routine/Geom/posOrigin_w ==
  x : Inport
  y : Inport  Port=2
  z : Inport  Port=3
  Frame1 : Concatenate  NumInputs=3  Mode=Multidimensional array  ConcatenateDimension=2
  Frame2 : Concatenate  NumInputs=3  Mode=Multidimensional array  ConcatenateDimension=2
  Subtract : Sum
  latOff : Constant  Value=MotoLatOfst
  longOff : Constant  Value=MotoLongOfst
  "vertOff " : Constant  Value=MotoVertOfst
  xyz : Outport
  wires:
  Subtract/1 -> xyz/1
  Frame2/1 -> Subtract/2
  longOff/1 -> Frame2/1
  "vertOff "/1 -> Frame2/3
  latOff/1 -> Frame2/2
  z/1 -> Frame1/3
  Frame1/1 -> Subtract/1
  x/1 -> Frame1/1
  y/1 -> Frame1/2

== system In_Plane_Model/Chassis, Tires, and Areo/Chassis Body, Suspension, and Steering/Signal routine/Geom/posRw_l ==
  x : Inport
  y : Inport  Port=2
  z : Inport  Port=3
  Frame1 : Concatenate  NumInputs=3  Mode=Multidimensional array  ConcatenateDimension=2
  xyz : Outport
  wires:
  y/1 -> Frame1/2
  x/1 -> Frame1/1
  z/1 -> Frame1/3
  Frame1/1 -> xyz/1

== system In_Plane_Model/Chassis, Tires, and Areo/Chassis Body, Suspension, and Steering/Signal routine/Info_sub/BdyFrm ==
  Fext_BF : Inport
  Fg : Inport  Port=2
  Fd : Inport  Port=3
  Md : Inport  Port=4
  Mext : Inport  Port=5
  Bus Creator7 : BusCreator  Inputs=4
  CG : Subsystem
  Forces : Subsystem
  Ground : Ground
  Moments : Subsystem
  F : PMIOPort  Side=Left
  seq : PMIOPort  Port=2  Side=Left
  BdyFrm : Outport
  wires:
  CG/1(Cg) -> Bus Creator7/1  "Cg"
  Mext/1 -> Moments/1(Mext)
  Moments/1(Moments) -> Bus Creator7/3  "Moments"
  Forces/1(Forces) -> Bus Creator7/2  "Forces"
  Fg/1 -> Forces/2(Fg)
  Bus Creator7/1 -> BdyFrm/1  "BdyFrm"
  Fd/1 -> Forces/3(Fd)
  Md/1 -> Moments/2(Md)
  Ground/1 -> Bus Creator7/4  "Pwr"
  Fext_BF/1 -> Forces/1(Fext_BF)
  connections:
  CG/LConn1 -- F/RConn1
  seq/RConn1 -- CG/LConn2

== system In_Plane_Model/Chassis, Tires, and Areo/Chassis Body, Suspension, and Steering/Signal routine/Info_sub/InertFrm ==
  Bus Creator : BusCreator  Inputs=1
  Convert to +Z down : Subsystem
  PS-Simulink Converter17 : nesl_utility/PS-Simulink Converter  PhysicalDomain=network_engine_domain  SubClassName=ps_output  LeftPortType=input  RightPortType=output  PseudoPeriodic=off  Frequencies=[]  VectorFormat=1-D array  Unit=m  AffineConversion=off
  PS-Simulink Converter19 : nesl_utility/PS-Simulink Converter  PhysicalDomain=network_engine_domain  SubClassName=ps_output  LeftPortType=input  RightPortType=output  PseudoPeriodic=off  Frequencies=[]  VectorFormat=1-D array  Unit=rad  AffineConversion=off
  PS-Simulink Converter25 : nesl_utility/PS-Simulink Converter  PhysicalDomain=network_engine_domain  SubClassName=ps_output  LeftPortType=input  RightPortType=output  PseudoPeriodic=off  Frequencies=[]  VectorFormat=1-D array  Unit=m  AffineConversion=off
  PS-Simulink Converter26 : nesl_utility/PS-Simulink Converter  PhysicalDomain=network_engine_domain  SubClassName=ps_output  LeftPortType=input  RightPortType=output  PseudoPeriodic=off  Frequencies=[]  VectorFormat=1-D array  Unit=m  AffineConversion=off
  PS-Simulink Converter27 : nesl_utility/PS-Simulink Converter  PhysicalDomain=network_engine_domain  SubClassName=ps_output  LeftPortType=input  RightPortType=output  PseudoPeriodic=off  Frequencies=[]  VectorFormat=1-D array  Unit=m/s  AffineConversion=off
  PS-Simulink Converter28 : nesl_utility/PS-Simulink Converter  PhysicalDomain=network_engine_domain  SubClassName=ps_output  LeftPortType=input  RightPortType=output  PseudoPeriodic=off  Frequencies=[]  VectorFormat=1-D array  Unit=m/s  AffineConversion=off
  PS-Simulink Converter29 : nesl_utility/PS-Simulink Converter  PhysicalDomain=network_engine_domain  SubClassName=ps_output  LeftPortType=input  RightPortType=output  PseudoPeriodic=off  Frequencies=[]  VectorFormat=1-D array  Unit=m/s  AffineConversion=off
  Transform Sensor Body : sm_lib/Frames and Transforms/Transform Sensor  MeasurementFrame=Base  RotationSequence=ZYX  SenseAngle=off  SenseAxis=off  SenseQ=off  SenseR=off  SenseRotationSequence=off  SenseOmegaX=off  SenseOmegaY=off  SenseOmegaZ=off  SenseOmega=off  SenseQDot=off  SenseRDot=off  SenseRotationSequenceDot=off  SenseAlphaX=off  SenseAlphaY=off  SenseAlphaZ=off  SenseAlpha=off  SenseQDDot=off  SenseRDDot=off  SenseX=on  SenseY=on  SenseZ=on  SenseXYZ=off  SenseRad=off  SenseAzim=off  SenseDist=off  SenseInc=off  SenseXDot=on  SenseYDot=on  SenseZDot=on  SenseXYZDot=off  SenseRadDot=off  SenseAzimDot=off  SenseDistDot=off  SenseIncDot=off  SenseXDDot=off  SenseYDDot=off  SenseZDDot=off  SenseXYZDDot=off  SenseRadDDot=off  SenseAzimDDot=off  SenseDistDDot=off  SenseIncDDot=off
  World Frame : sm_lib/Frames and Transforms/World Frame
  X+pi : sm_lib/Frames and Transforms/Rigid Transform  RotationMethod=StandardAxis  FollAlignAxisA=+X  BaseAlignAxisA=+Y  FollAlignAxisB=+Y  BaseAlignAxisB=+Z  RotationStandardAxis=+X  RotationAngle=pi  RotationAngleUnits=rad  RotationArbitraryAxis=[0 0 1]  RotationSequenceAxes=FollowerAxes  RotationSequence=XYX  RotationSequenceAngles=[0 0 0]  RotationSequenceAnglesUnits=deg  RotationMatrix=[1 0 0; 0 1 0; 0 0 1]  Quaternion=[1 0 0 0]  TranslationMethod=None  TranslationCartesianOffset=[0 0 0]  TranslationCartesianOffsetUnits=m  TranslationStandardAxis=+Z  TranslationStandardOffset=0  TranslationStandardOffsetUnits=m  TranslationROffset=0  TranslationROffsetUnits=m  TranslationThetaOffset=0  TranslationThetaOffsetUnits=deg  TranslationZOffset=0  TranslationZOffsetUnits=m
  seq : PMIOPort  Side=Left
  CG : PMIOPort  Port=2  Side=Left
  InertFrm : Outport
  wires:
  Bus Creator/1 -> InertFrm/1  "InertFrm"
  PS-Simulink Converter19/1 -> Convert to +Z down/1(seq)  "seq"
  PS-Simulink Converter27/1 -> Convert to +Z down/5(Xdot)  "Xdot"
  PS-Simulink Converter17/1 -> Convert to +Z down/2(X)  "X"
  PS-Simulink Converter25/1 -> Convert to +Z down/3(Y)  "Y"
  PS-Simulink Converter28/1 -> Convert to +Z down/6(Ydot)  "Ydot"
  PS-Simulink Converter26/1 -> Convert to +Z down/4(Z)  "Z"
  PS-Simulink Converter29/1 -> Convert to +Z down/7(Zdot)  "Zdot"
  Convert to +Z down/1(Cg) -> Bus Creator/1  "Cg"
  connections:
  Transform Sensor Body/RConn1 -- CG/RConn1
  PS-Simulink Converter28/LConn1 -- Transform Sensor Body/RConn6
  PS-Simulink Converter29/LConn1 -- Transform Sensor Body/RConn7
  PS-Simulink Converter25/LConn1 -- Transform Sensor Body/RConn3
  Transform Sensor Body/RConn4 -- PS-Simulink Converter26/LConn1
  Transform Sensor Body/RConn5 -- PS-Simulink Converter27/LConn1
  Transform Sensor Body/RConn2 -- PS-Simulink Converter17/LConn1
  World Frame/RConn1 -- X+pi/LConn1
  seq/RConn1 -- PS-Simulink Converter19/LConn1
  X+pi/RConn1 -- Transform Sensor Body/LConn1

== system In_Plane_Model/Chassis, Tires, and Areo/Tire/Front Tire/Linear Front SSC Tire/Brake model ==
  BrkPrs : Inport
  Omega : Inport  Port=2
  MBrkin : Inport  Port=3
  External : Subsystem  VariantControl=External
  MW Brake : Subsystem  VariantControl=MW Brake
  MBrk : Outport

== system In_Plane_Model/Chassis, Tires, and Areo/Tire/Front Tire/Linear Front SSC Tire/Contact model ==
  rz : Inport
  pz : Inport  Port=2
  Fzin : Inport  Port=3
  External : Subsystem  VariantControl=External
  Simple spring and damper : Subsystem  VariantControl=Simple spring and damper
  Fz : Outport

== system In_Plane_Model/Chassis, Tires, and Areo/Tire/Front Tire/Linear Front SSC Tire/Friction model ==
  rx : Inport
  ry : Inport  Port=2
  rz : Inport  Port=3
  Fz : Inport  Port=4
  Omega : Inport  Port=5
  A,V,P_WhlRoll : Inport  Port=6
  Fxin : Inport  Port=7
  Fyin : Inport  Port=8
  Mxin : Inport  Port=9
  Myin : Inport  Port=10
  Mzin : Inport  Port=11
  External : Subsystem  VariantControl=External
  Linear : Subsystem  VariantControl=Linear
  Fx : Outport
  Fy : Outport  Port=2
  Mx : Outport  Port=3
  My : Outport  Port=4
  Mz : Outport  Port=5
  Kappa : Outport  Port=6
  Alpha : Outport  Port=7

== system In_Plane_Model/Chassis, Tires, and Areo/Tire/Front Tire/Linear Front SSC Tire/Simscape ==
  MWh : Inport
  Mbrk : Inport  Port=2
  Mcr : Inport  Port=3
  Fx : Inport  Port=4
  Fy : Inport  Port=5
  Fz : Inport  Port=6
  Mxin : Inport  Port=7
  Myin : Inport  Port=8
  Mzin : Inport  Port=9
  Reaction Torque : Subsystem
  Sensor : Subsystem
  Simscape Multibody Rim&Wheel : Subsystem
  apply forces and moments : Subsystem
  B : PMIOPort  Side=Left
  M : PMIOPort  Port=2  Side=Left
  omega : Outport
  omegadot : Outport  Port=2
  Info_CP : Outport  Port=3
  A,V,P_WhlRoll : Outport  Port=4
  rx : Outport  Port=5
  ry : Outport  Port=6
  rz : Outport  Port=7
  pz : Outport  Port=8
  wires:
  Simscape Multibody Rim&Wheel/4(Info_CP) -> Info_CP/1
  Fx/1 -> Simscape Multibody Rim&Wheel/2(Fx), apply forces and moments/1(Fx)
  MWh/1 -> Reaction Torque/1(MWh), Simscape Multibody Rim&Wheel/1(MWh)
  Simscape Multibody Rim&Wheel/1(omega) -> omega/1
  Mbrk/1 -> Reaction Torque/2(Mbrk), Simscape Multibody Rim&Wheel/3(Mbrk)
  Mcr/1 -> Simscape Multibody Rim&Wheel/4(Mcr)
  Sensor/1(rx) -> rx/1
  Sensor/4(pz) -> pz/1
  Simscape Multibody Rim&Wheel/3(A,V,P_WhlRoll) -> A,V,P_WhlRoll/1
  Fz/1 -> apply forces and moments/3(Fz)
  Sensor/2(ry) -> ry/1
  Fy/1 -> apply forces and moments/2(Fy)
  Sensor/3(rz) -> rz/1
  Mxin/1 -> apply forces and moments/4(Mxin)
  Mzin/1 -> apply forces and moments/5(Mzin)
  Myin/1 -> Simscape Multibody Rim&Wheel/5(Myin)
  Simscape Multibody Rim&Wheel/2(omegadot) -> omegadot/1
  connections:
  Reaction Torque/RConn1 -- M/RConn1
  Simscape Multibody Rim&Wheel/RConn1 -- Sensor/LConn1 -- apply forces and moments/RConn1
  B/RConn1 -- Simscape Multibody Rim&Wheel/LConn1

== system In_Plane_Model/Chassis, Tires, and Areo/Tire/Rear Tire/Linear Rear SSC Tire/Brake model ==
  BrkPrs : Inport
  Omega : Inport  Port=2
  MBrkin : Inport  Port=3
  External : Subsystem  VariantControl=External
  MW Brake : Subsystem  VariantControl=MW Brake
  MBrk : Outport

== system In_Plane_Model/Chassis, Tires, and Areo/Tire/Rear Tire/Linear Rear SSC Tire/Contact model ==
  rz : Inport
  pz : Inport  Port=2
  Fzin : Inport  Port=3
  External : Subsystem  VariantControl=External
  Simple spring and damper : Subsystem  VariantControl=Simple spring and damper
  Fz : Outport

== system In_Plane_Model/Chassis, Tires, and Areo/Tire/Rear Tire/Linear Rear SSC Tire/Friction model ==
  rx : Inport
  ry : Inport  Port=2
  rz : Inport  Port=3
  Fz : Inport  Port=4
  Omega : Inport  Port=5
  A,V,P_WhlRoll : Inport  Port=6
  Fxin : Inport  Port=7
  Fyin : Inport  Port=8
  Mxin : Inport  Port=9
  Myin : Inport  Port=10
  Mzin : Inport  Port=11
  External : Subsystem  VariantControl=External
  Linear : Subsystem  VariantControl=Linear
  Fx : Outport
  Fy : Outport  Port=2
  Mx : Outport  Port=3
  My : Outport  Port=4
  Mz : Outport  Port=5
  Kappa : Outport  Port=6
  Alpha : Outport  Port=7
